simulink model "for_nonparametric_identification"  (R2023a)
settings: Solver=VariableStepAuto  StartTime=0.0  StopTime=150  RelTol=1e-3
values from neighbouring files (symbols this model uses):
  Ts = 0.1    [main.m]
settings Model: Creator=Gasper  LastModifiedBy=Gasper

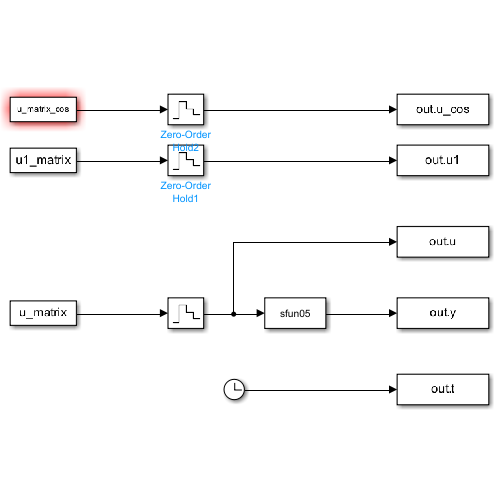
[thumbnail: Simulink's stored preview of the top-level diagram]
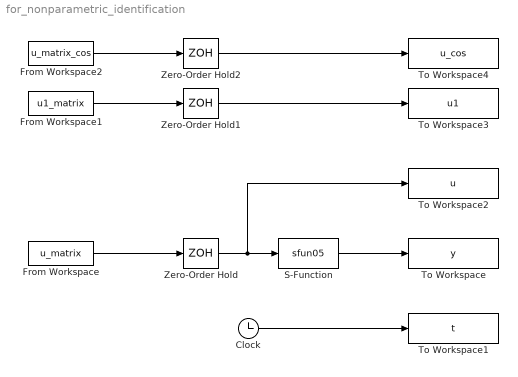
== system for_nonparametric_identification ==
  Clock : Clock
  From Workspace : FromWorkspace  VariableName=u_matrix  SampleTime=Ts
  From Workspace1 : FromWorkspace  VariableName=u1_matrix  SampleTime=Ts
  From Workspace2 : FromWorkspace  VariableName=u_matrix_cos  SampleTime=Ts
  S-Function : S-Function  FunctionName=sfun05  SFunctionDeploymentMode=off  EnableBusSupport=off
  To Workspace : ToWorkspace  VariableName=y  SaveFormat=Timeseries  SampleTime=Ts
  To Workspace1 : ToWorkspace  VariableName=t  SaveFormat=Timeseries  SampleTime=Ts
  To Workspace2 : ToWorkspace  VariableName=u  SaveFormat=Timeseries  SampleTime=Ts
  To Workspace3 : ToWorkspace  VariableName=u1  SaveFormat=Timeseries  SampleTime=Ts
  To Workspace4 : ToWorkspace  VariableName=u_cos  SaveFormat=Timeseries  SampleTime=Ts
  Zero-Order Hold : ZeroOrderHold  SampleTime=Ts
  Zero-Order Hold1 : ZeroOrderHold  SampleTime=Ts
  Zero-Order Hold2 : ZeroOrderHold  SampleTime=Ts
  wires:
  Zero-Order Hold/1 -> To Workspace2/1, S-Function/1
  From Workspace/1 -> Zero-Order Hold/1
  Clock/1 -> To Workspace1/1
  S-Function/1 -> To Workspace/1
  From Workspace1/1 -> Zero-Order Hold1/1
  Zero-Order Hold1/1 -> To Workspace3/1
  From Workspace2/1 -> Zero-Order Hold2/1
  Zero-Order Hold2/1 -> To Workspace4/1
